simulink model "simulink_controll_altitude_5kg"  (R2015a)
settings: Solver=ode45  StartTime=0.0  StopTime=10.0  RelTol=1e-3
libraries: fuzblock x2
settings Model: Creator=Marcos  LastModifiedBy=Marcos

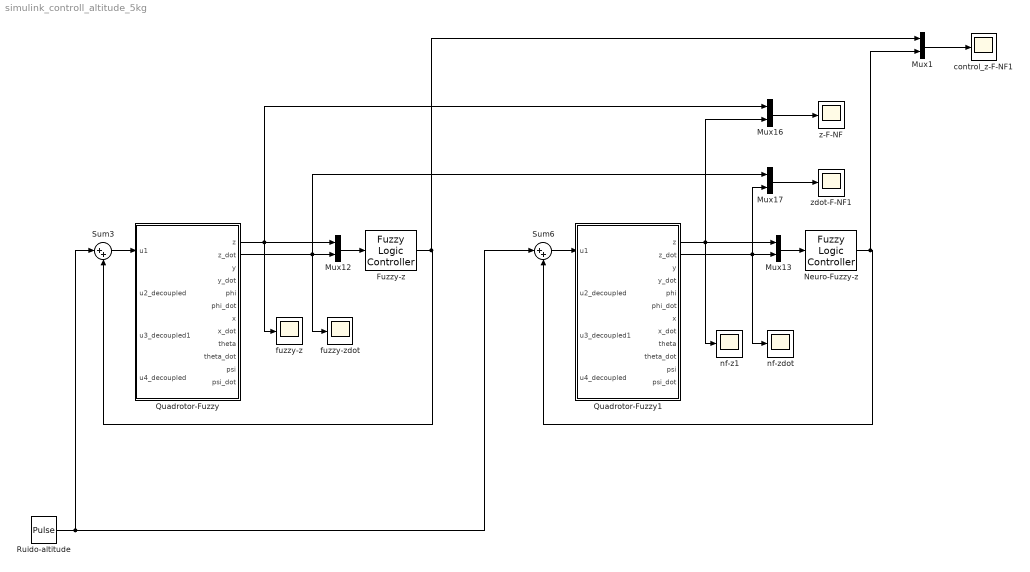
== system simulink_controll_altitude_5kg ==
  Fuzzy-z : fuzblock/Fuzzy Logic  Controller  fis='fis_altitude.fis'
  Mux{1,12..13,16..17} (5 alike) : Mux  Inputs=2
  Neuro-Fuzzy-z : fuzblock/Fuzzy Logic  Controller  fis='anfis_altitude.fis'
  Quadrotor-Fuzzy : Subsystem
  Quadrotor-Fuzzy1 : Subsystem
  Ruido-altitude : DiscretePulseGenerator  PulseType=Time based  Amplitude=100  Period=10
  Sum3 : Sum  Inputs=|++
  Sum6 : Sum  Inputs=|++
  control_z-F-NF1 : Scope
      settings: SaveName=control_z5
  fuzzy-z : Scope
      settings: SaveName=ScopeData17
  fuzzy-zdot : Scope
      settings: SaveName=ScopeData18
  nf-z1 : Scope
      settings: SaveName=ScopeData23
  nf-zdot : Scope
      settings: SaveName=ScopeData24
  z-F-NF : Scope
      settings: SaveName=z5
  zdot-F-NF1 : Scope
      settings: SaveName=zdot5
  wires:
  Mux12/1 -> Fuzzy-z/1
  Fuzzy-z/1 -> Mux1/1, Sum3/2
  Sum3/1 -> Quadrotor-Fuzzy/1(u1)
  Quadrotor-Fuzzy/1(z) -> Mux16/1, fuzzy-z/1, Mux12/1
  Quadrotor-Fuzzy/2(z_dot) -> Mux17/1, fuzzy-zdot/1, Mux12/2
  Mux13/1 -> Neuro-Fuzzy-z/1
  Ruido-altitude/1 -> Sum3/1, Sum6/1
  Neuro-Fuzzy-z/1 -> Mux1/2, Sum6/2
  Sum6/1 -> Quadrotor-Fuzzy1/1(u1)
  Quadrotor-Fuzzy1/1(z) -> Mux16/2, nf-z1/1, Mux13/1
  Quadrotor-Fuzzy1/2(z_dot) -> Mux17/2, nf-zdot/1, Mux13/2
  Mux16/1 -> z-F-NF/1
  Mux17/1 -> zdot-F-NF1/1
  Mux1/1 -> control_z-F-NF1/1

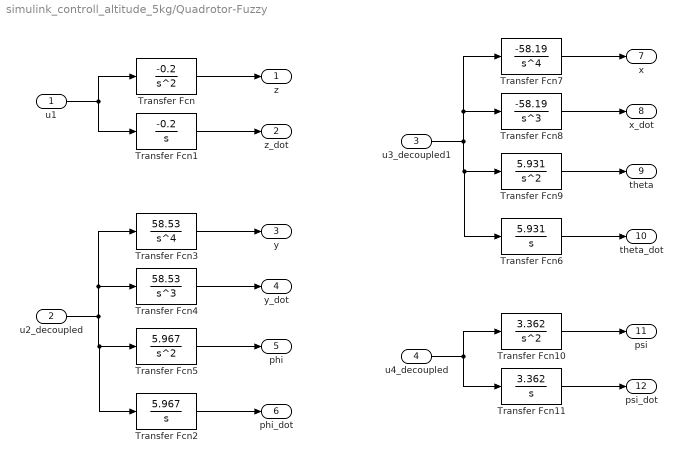
== system simulink_controll_altitude_5kg/Quadrotor-Fuzzy ==
  u1 : Inport
  u2_decoupled : Inport  Port=2
  u3_decoupled1 : Inport  Port=3
  u4_decoupled : Inport  Port=4
  Transfer Fcn : TransferFcn  Numerator=[-0.2]  Denominator=[1 0 0]
  Transfer Fcn1 : TransferFcn  Numerator=[-0.2]  Denominator=[1 0]
  Transfer Fcn10 : TransferFcn  Numerator=[3.362]  Denominator=[1 0 0]
  Transfer Fcn11 : TransferFcn  Numerator=[3.362]  Denominator=[1 0]
  Transfer Fcn2 : TransferFcn  Numerator=[5.967]  Denominator=[1 0]
  Transfer Fcn3 : TransferFcn  Numerator=[58.53]  Denominator=[1 0 0 0 0]
  Transfer Fcn4 : TransferFcn  Numerator=[58.53]  Denominator=[1 0 0 0]
  Transfer Fcn5 : TransferFcn  Numerator=[5.967]  Denominator=[1 0 0]
  Transfer Fcn6 : TransferFcn  Numerator=[5.931]  Denominator=[1 0]
  Transfer Fcn7 : TransferFcn  Numerator=[-58.19]  Denominator=[1 0 0 0 0]
  Transfer Fcn8 : TransferFcn  Numerator=[-58.19]  Denominator=[1 0 0 0]
  Transfer Fcn9 : TransferFcn  Numerator=[5.931]  Denominator=[1 0 0]
  z : Outport
  z_dot : Outport  Port=2
  y : Outport  Port=3
  y_dot : Outport  Port=4
  phi : Outport  Port=5
  phi_dot : Outport  Port=6
  x : Outport  Port=7
  x_dot : Outport  Port=8
  theta : Outport  Port=9
  theta_dot : Outport  Port=10
  psi : Outport  Port=11
  psi_dot : Outport  Port=12
  wires:
  Transfer Fcn/1 -> z/1
  u1/1 -> Transfer Fcn/1, Transfer Fcn1/1
  Transfer Fcn1/1 -> z_dot/1
  Transfer Fcn3/1 -> y/1
  u2_decoupled/1 -> Transfer Fcn3/1, Transfer Fcn4/1, Transfer Fcn2/1, Transfer Fcn5/1
  Transfer Fcn4/1 -> y_dot/1
  Transfer Fcn5/1 -> phi/1
  Transfer Fcn2/1 -> phi_dot/1
  Transfer Fcn7/1 -> x/1
  u3_decoupled1/1 -> Transfer Fcn7/1, Transfer Fcn8/1, Transfer Fcn6/1, Transfer Fcn9/1
  Transfer Fcn8/1 -> x_dot/1
  Transfer Fcn9/1 -> theta/1
  Transfer Fcn6/1 -> theta_dot/1
  Transfer Fcn10/1 -> psi/1
  u4_decoupled/1 -> Transfer Fcn10/1, Transfer Fcn11/1
  Transfer Fcn11/1 -> psi_dot/1

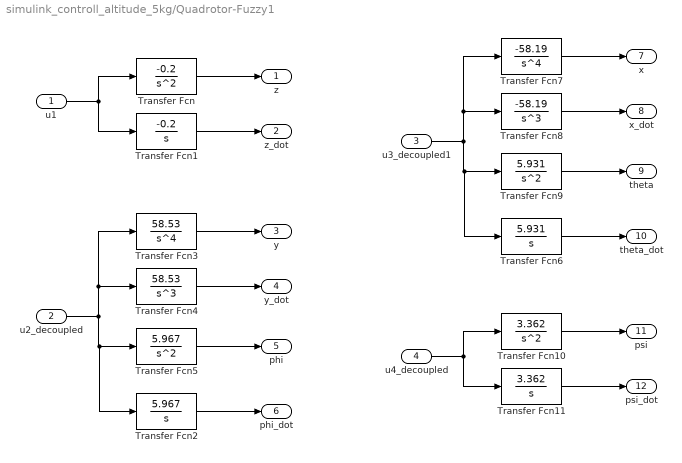
== system simulink_controll_altitude_5kg/Quadrotor-Fuzzy1 ==
  u1 : Inport
  u2_decoupled : Inport  Port=2
  u3_decoupled1 : Inport  Port=3
  u4_decoupled : Inport  Port=4
  Transfer Fcn : TransferFcn  Numerator=[-0.2]  Denominator=[1 0 0]
  Transfer Fcn1 : TransferFcn  Numerator=[-0.2]  Denominator=[1 0]
  Transfer Fcn10 : TransferFcn  Numerator=[3.362]  Denominator=[1 0 0]
  Transfer Fcn11 : TransferFcn  Numerator=[3.362]  Denominator=[1 0]
  Transfer Fcn2 : TransferFcn  Numerator=[5.967]  Denominator=[1 0]
  Transfer Fcn3 : TransferFcn  Numerator=[58.53]  Denominator=[1 0 0 0 0]
  Transfer Fcn4 : TransferFcn  Numerator=[58.53]  Denominator=[1 0 0 0]
  Transfer Fcn5 : TransferFcn  Numerator=[5.967]  Denominator=[1 0 0]
  Transfer Fcn6 : TransferFcn  Numerator=[5.931]  Denominator=[1 0]
  Transfer Fcn7 : TransferFcn  Numerator=[-58.19]  Denominator=[1 0 0 0 0]
  Transfer Fcn8 : TransferFcn  Numerator=[-58.19]  Denominator=[1 0 0 0]
  Transfer Fcn9 : TransferFcn  Numerator=[5.931]  Denominator=[1 0 0]
  z : Outport
  z_dot : Outport  Port=2
  y : Outport  Port=3
  y_dot : Outport  Port=4
  phi : Outport  Port=5
  phi_dot : Outport  Port=6
  x : Outport  Port=7
  x_dot : Outport  Port=8
  theta : Outport  Port=9
  theta_dot : Outport  Port=10
  psi : Outport  Port=11
  psi_dot : Outport  Port=12
  wires:
  Transfer Fcn/1 -> z/1
  u1/1 -> Transfer Fcn/1, Transfer Fcn1/1
  Transfer Fcn1/1 -> z_dot/1
  Transfer Fcn3/1 -> y/1
  u2_decoupled/1 -> Transfer Fcn3/1, Transfer Fcn4/1, Transfer Fcn2/1, Transfer Fcn5/1
  Transfer Fcn4/1 -> y_dot/1
  Transfer Fcn5/1 -> phi/1
  Transfer Fcn2/1 -> phi_dot/1
  Transfer Fcn7/1 -> x/1
  u3_decoupled1/1 -> Transfer Fcn7/1, Transfer Fcn8/1, Transfer Fcn6/1, Transfer Fcn9/1
  Transfer Fcn8/1 -> x_dot/1
  Transfer Fcn9/1 -> theta/1
  Transfer Fcn6/1 -> theta_dot/1
  Transfer Fcn10/1 -> psi/1
  u4_decoupled/1 -> Transfer Fcn10/1, Transfer Fcn11/1
  Transfer Fcn11/1 -> psi_dot/1
